simulink model "Inputs"  (R2020a)
settings: Solver=FixedStepAuto  StartTime=0.0  StopTime=10.0  FixedStep=1e-3  RelTol=1e-3  EnableMultiTasking=on
undefined symbols (not defined in the file): A1, D0, D1, D10, D11, D12, D13, D2, D3, D4, D5, D6, D7, D8, D9, PTA0, PTA1, PTA2, PTB23, PTB3, PTB9, PTC16, PTC17, PTC2, PTC3, PTC4, PTD0, PTD1, PTD2, PTD3
libraries: frdmk64flib x18
settings Model: ExtModeTrigDuration=5  Creator=WinnieTrandinh  LastModifiedBy=WinnieTrandinh
settings OptimizationCC: EnhancedBackFolding=on  PassReuseOutputArgsAs=Individual arguments  ZeroExternalMemoryAtStartup=off  ZeroInternalMemoryAtStartup=off  MaxStackSize=64  OptimizeBlockOrder=speed  DifferentSizesBufferReuse=on  OptimizationCustomize=off  EfficientTunableParamExpr=on
settings DebuggingCC: ParameterTunabilityLossMsg=error
settings HardwareCC: ProdBitPerPointer=32  ProdBitPerSizeT=32  ProdBitPerPtrDiffT=32  ProdLargestAtomicInteger=Long  ProdLargestAtomicFloat=Double  ProdWordSize=32  ProdHWDeviceType=ARM Compatible->ARM Cortex
settings SFSimCC: MATLABDynamicMemAlloc=off
settings RTWCC: SystemTargetFile=ert.tlc  HardwareBoard=NXP FRDM-K64F  TemplateMakefile=ert_default_tmf  Toolchain=GNU Tools for ARM Embedded Processors
settings CodeAppCC: ForceParamTrailComments=on  IgnoreCustomStorageClasses=off  OperatorAnnotations=on  SimulinkDataObjDesc=on  SFDataObjDesc=on  InsertBlockDesc=on

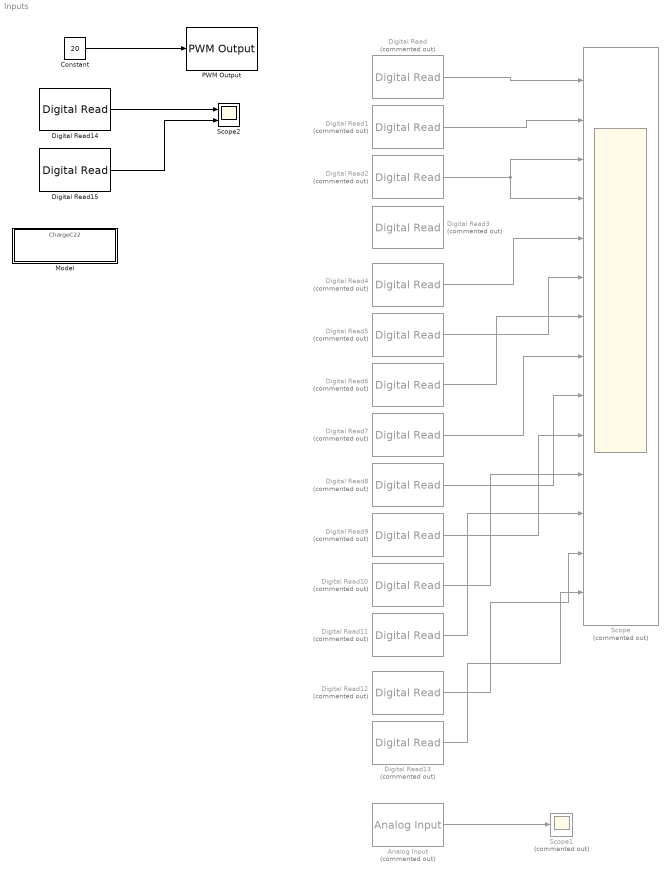
== system Inputs ==
  Analog Input : frdmk64flib/Analog Input  Commented=on  Whichpin=PTB3 (A1)  SampleTime=-1
  Constant : Constant  Value=20
  Digital Read : frdmk64flib/Digital Read  Commented=on  Whichpin=PTC16 (D0)  SampleTime=-1
  Digital Read1 : frdmk64flib/Digital Read  Commented=on  Whichpin=PTC17 (D1)  SampleTime=-1
  Digital Read10 : frdmk64flib/Digital Read  Commented=on  Whichpin=PTD0 (D10)  SampleTime=-1
  Digital Read11 : frdmk64flib/Digital Read  Commented=on  Whichpin=PTD2 (D11)  SampleTime=-1
  Digital Read12 : frdmk64flib/Digital Read  Commented=on  Whichpin=PTD3 (D12)  SampleTime=-1
  Digital Read13 : frdmk64flib/Digital Read  Commented=on  Whichpin=PTD1 (D13)  SampleTime=-1
  Digital Read14 : frdmk64flib/Digital Read  Whichpin=PTC17 (D1)  SampleTime=-1
  Digital Read15 : frdmk64flib/Digital Read  Whichpin=PTC16 (D0)  SampleTime=-1
  Digital Read2 : frdmk64flib/Digital Read  Commented=on  Whichpin=PTB9 (D2)  SampleTime=-1
  Digital Read3 : frdmk64flib/Digital Read  Commented=on  Whichpin=PTA1 (D3)  SampleTime=-1
  Digital Read4 : frdmk64flib/Digital Read  Commented=on  Whichpin=PTB23 (D4)  SampleTime=-1
  Digital Read5 : frdmk64flib/Digital Read  Commented=on  Whichpin=PTA2 (D5)  SampleTime=-1
  Digital Read6 : frdmk64flib/Digital Read  Commented=on  Whichpin=PTC2 (D6)  SampleTime=-1
  Digital Read7 : frdmk64flib/Digital Read  Commented=on  Whichpin=PTC3 (D7)  SampleTime=-1
  Digital Read8 : frdmk64flib/Digital Read  Commented=on  Whichpin=PTA0 (D8)  SampleTime=-1
  Digital Read9 : frdmk64flib/Digital Read  Commented=on  Whichpin=PTC4 (D9)  SampleTime=-1
  Model : ModelReference  ModelNameDialog=ChargeC22.slx  SimulationMode=Normal  ModelReferenceVersion=1.6
  PWM Output : frdmk64flib/PWM Output  Whichpin=PTC2 (D6)  InitialFrequency=2000  InitialDutyCycle=20
  Scope : Scope  Commented=on  NumInputPorts=14
  Scope1 : Scope  Commented=on
  Scope2 : Scope  NumInputPorts=2
  wires:
  Digital Read/1 -> Scope/1
  Digital Read1/1 -> Scope/2
  Digital Read2/1 -> Scope/4, Scope/3
  Digital Read7/1 -> Scope/8
  Digital Read6/1 -> Scope/7
  Digital Read4/1 -> Scope/5
  Digital Read5/1 -> Scope/6
  Digital Read9/1 -> Scope/10
  Digital Read8/1 -> Scope/9
  Digital Read10/1 -> Scope/11
  Digital Read11/1 -> Scope/12
  Digital Read13/1 -> Scope/14
  Digital Read12/1 -> Scope/13
  Constant/1 -> PWM Output/1
  Analog Input/1 -> Scope1/1
  Digital Read14/1 -> Scope2/1
  Digital Read15/1 -> Scope2/2
